simulink model "open_loop_tank"  (Simulink 10.0)
settings: Solver=ode45  StartTime=0.0  StopTime=199.99  MaxStep=0.1  RelTol=1e-3  EnableMultiTasking=on
libraries: simulink x1
settings Model: Creator=akari  LastModifiedBy=linesLK
settings DataIOCC: LimitDataPoints=on  MaxDataPoints=10000  SignalLoggingSaveFormat=ModelDataLogs
settings OptimizationCC: ExpressionDepthLimit=2147483647
settings DebuggingCC: SolverPrmCheckMsg=warning  FcnCallInpInsideContextMsg=warning  StateNameClashWarn=warning
settings GRTTargetCC: GeneratePreprocessorConditionals=Disable all
settings ConfigComp: CovExternalEMLEnable=off

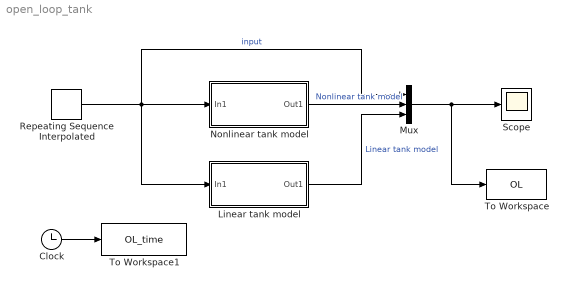
== system open_loop_tank ==
  Clock : Clock
  Linear tank model : Subsystem
  Mux : Mux  Inputs=3
  Nonlinear tank model : Subsystem
  Repeating Sequence Interpolated : simulink/Sources/Repeating Sequence Interpolated  OutValues=[0.4 0.6 0.3 0.7]  TimeValues=[0 40 80 120]  LookUpMeth=Interpolation-Use End Values  tsamp=-1  OutMin=[]  OutMax=[]  OutDataTypeStr=double  OutputDataTypeScalingMode=double  OutDataType=double  OutScaling=2^-10
  Scope : Scope
  To Workspace : ToWorkspace  VariableName=OL  SampleTime=-1
  To Workspace1 : ToWorkspace  VariableName=OL_time  SampleTime=-1
  wires:
  Mux/1 -> Scope/1, To Workspace/1
  Nonlinear tank model/1(Out1) -> Mux/2  "Nonlinear tank model"
  Linear tank model/1(Out1) -> Mux/3  "Linear tank model"
  Repeating Sequence Interpolated/1 -> Nonlinear tank model/1(In1), Linear tank model/1(In1), Mux/1  "input"
  Clock/1 -> To Workspace1/1

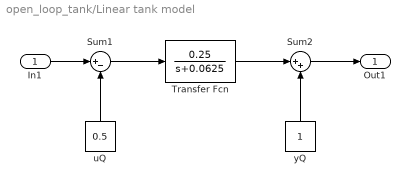
== system open_loop_tank/Linear tank model ==
  In1 : Inport
  Sum1 : Sum  Inputs=|+-
  Sum2 : Sum  Inputs=|++
  Transfer Fcn : TransferFcn  Numerator=[0.25]  Denominator=[1 0.0625]
  uQ : Constant  Value=0.5
  yQ : Constant
  Out1 : Outport
  wires:
  Sum1/1 -> Transfer Fcn/1
  Transfer Fcn/1 -> Sum2/1
  yQ/1 -> Sum2/2
  uQ/1 -> Sum1/2
  Sum2/1 -> Out1/1
  In1/1 -> Sum1/1

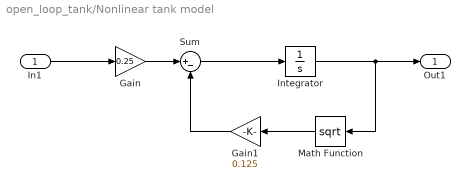
== system open_loop_tank/Nonlinear tank model ==
  In1 : Inport
  Gain : Gain  Gain=0.25
  Gain1 : Gain  Gain=0.125
  Integrator : Integrator  InitialCondition=1
  Math Function : Math  Operator=sqrt  SaturateOnIntegerOverflow=on
  Sum : Sum  Inputs=|+-
  Out1 : Outport
  wires:
  Sum/1 -> Integrator/1
  Integrator/1 -> Math Function/1, Out1/1
  Math Function/1 -> Gain1/1
  Gain/1 -> Sum/1
  Gain1/1 -> Sum/2
  In1/1 -> Gain/1
